simulink model "PubIfDecisionVSM_ESS"  (R2020b)
settings: Solver=FixedStepAuto  StartTime=0.0  StopTime=Inf  RelTol=1e-3
PostLoadFcn:
  | if any(exist('dsrtsu_mdlpostloadfcn', 'file') ~= 0), dsrtsu_mdlpostloadfcn('Execute', bdroot); end
InitFcn:
  | , if any(exist('rtifpga_mdlclblib', 'file') ~= 0), rtifpga_mdlclblib('Init', bdroot); end,
  | , if any(exist('dsmpb_private', 'file') ~= 0), dsmpb_private('dsmpb_mdlclblib', 'Init', bdroot); end,
PreSaveFcn:
  | , if any(exist('dsmpb_private', 'file') ~= 0), dsmpb_private('dsmpb_mdlclblib', 'PreSave', bdroot); end,
CloseFcn:
  | , if any(exist('dsmpb_private', 'file') ~= 0), dsmpb_private('dsmpb_mdlclblib', 'Close', bdroot); end,
settings Model: DataDictionary=HWA_DDs.sldd  RTICANMMDATA=struct('GeneralSetupData',struct('modelroot','E:\System\ADAS_BaseModel\ADAS_Store\Adas\VSM\ESS','generalsettings',struct('filesettings',struct('destfolder',struct('Name','RTICANMM_FILES','Check',1),'buildfolder',struct('Name','.','Check',1),'AbsDestfolder',struct('Name','E:\System\ADAS_BaseModel\ADAS_Store\Adas\VSM\ESS\RTICANMM_FILES'),'AbsBuildfolder',struct('Name','E:\System\ADAS_BaseModel\ADAS_Store\Adas\VSM\ESS'))),'options',struct('addpaths',1,'rmpaths',1,'addtrcexclusion',false,'cannavigator',struct('checkmonitoring',0),'show_usrtrc',0,'use_usrtrc',0),'advanced',struct('options',ones(1,100)),'MPSetup',{{}},'RTI',struct('Type','DSRT','Ver','4.4','Date','02-Nov-2020'),'modelname','PubIfDecisionVSM_ESS','block','PubIfDecisionVSM_ESS'))  DSRTSU_INTERNAL_RTIFPGA=170  Creator=GW00180895  LastModifiedBy=GW00164938
settings OptimizationCC: BlockReduction=off  ConditionallyExecuteInputs=off  OptimizeBlockIOStorage=off  BufferReuse=off  GlobalBufferReuse=off  ExpressionFolding=off  LocalBlockOutputs=off  OptimizeDataStoreBuffers=off  BusAssignmentInplaceUpdate=off
settings DebuggingCC: TasksWithSamePriorityMsg=none
settings HardwareCC: ProdBitPerPointer=32  ProdBitPerSizeT=32  ProdBitPerPtrDiffT=32  ProdLargestAtomicInteger=Integer  ProdWordSize=32  ProdHWDeviceType=Custom Processor->Custom
settings ModelReferenceCC: UpdateModelReferenceTargets=IfOutOfDate  EnableParallelModelReferenceBuilds=on  ModelReferenceNumInstancesAllowed=Single
settings SFSimCC: MATLABDynamicMemAlloc=off
settings RTWCC: Description=dSPACE Run-Time Target (for VEOS on Windows and ConfigurationDesk)  SystemTargetFile=dsrt.tlc  GenCodeOnly=on  MakeCommand=make_dsrt  TemplateMakefile=dsrt_default_tmf  RTWVerbose=off
settings STFCustomTargetCC: TargetLangStandard=C99 (ISO)  ParMdlRefBuildCompliant=on  ConcurrentExecutionCompliant=off  CPPClassGenCompliant=off  GRTInterface=off  SystemTargetFile=dsrt.tlc
settings GRTTargetCC: CompOptLevelCompliant=off  ConcurrentExecutionCompliant=off  CombineOutputUpdateFcns=off  MatFileLogging=off  CPPClassGenCompliant=off  UseToolchainInfoCompliant=off

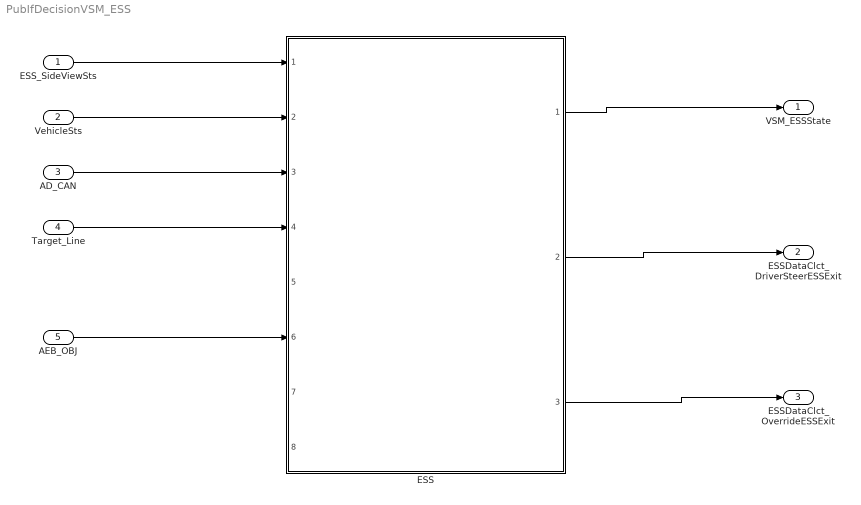
== system PubIfDecisionVSM_ESS ==
  ESS_SideViewSts : Inport  OutDataTypeStr=Bus: PLAN_DPC_ESS_BUS
  VehicleSts : Inport  Port=2  OutDataTypeStr=Bus: ESS_VehicleSts_BUS
  AD_CAN : Inport  Port=3  OutDataTypeStr=Bus: ESS_AD_CAN_BUS
  Target_Line : Inport  Port=4  OutDataTypeStr=Bus: LSM_ESS_BUS
  AEB_OBJ : Inport  Port=5  OutDataTypeStr=Bus: TOS_AEB_LONOBJ_BUS
  ESS : Subsystem  ReferencedSubsystem=PvtSubSys_VSM_ESS
  VSM_ESSState : Outport
  ESSDataClct_DriverSteerESSExit : Outport  Port=2
  ESSDataClct_OverrideESSExit : Outport  Port=3
  wires:
  Target_Line/1 -> ESS/4
  AD_CAN/1 -> ESS/3
  AEB_OBJ/1 -> ESS/6
  VehicleSts/1 -> ESS/2
  ESS_SideViewSts/1 -> ESS/1
  ESS/2 -> ESSDataClct_DriverSteerESSExit/1
  ESS/3 -> ESSDataClct_OverrideESSExit/1
  ESS/1 -> VSM_ESSState/1
